simulink subsystem "EoM_Euler6DoF"  (R2024b)
settings: Solver=VariableStepAuto  StartTime=0.0  StopTime=10.0  RelTol=1e-3
undefined symbols (not defined in the file or in its folder): com_error, inertia_error, mass_error, vehicle
settings Model: Creator=thatf  LastModifiedBy=ishkr

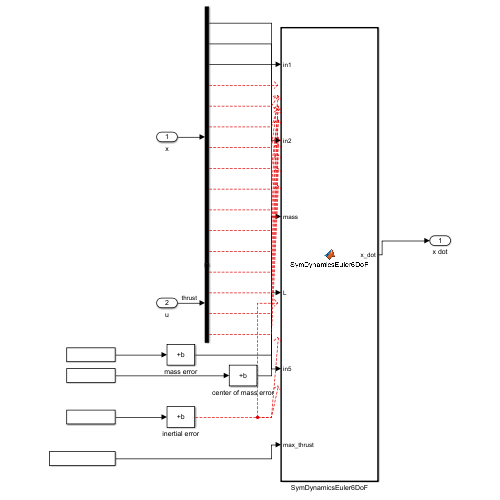
[thumbnail: Simulink's stored preview of the top-level diagram]
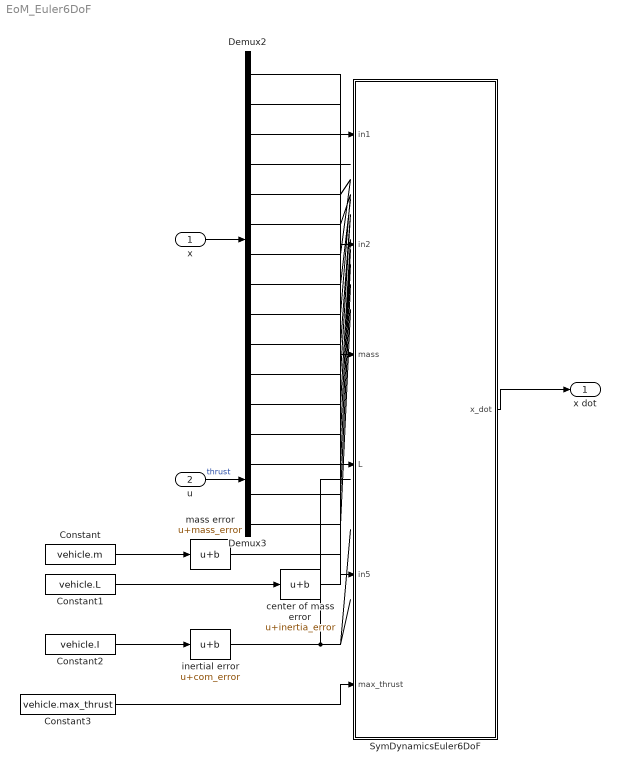
== system EoM_Euler6DoF ==
  x : Inport
  u : Inport  Port=2
  Constant : Constant  Value=vehicle.m
  Constant1 : Constant  Value=vehicle.L
  Constant2 : Constant  Value=vehicle.I
  Constant3 : Constant  Value=vehicle.max_thrust
  Demux2 : Demux  Outputs=dof.nx
  Demux3 : Demux  Outputs=dof.nu
  SymDynamicsEuler6DoF : MATLAB Function  TreatAsAtomicUnit=on
  center of mass error : Bias  Bias=inertia_error  SaturateOnIntegerOverflow=off
  inertial error : Bias  Bias=com_error  SaturateOnIntegerOverflow=off
  mass error : Bias  Bias=mass_error  SaturateOnIntegerOverflow=off
  x dot : Outport
  wires:
  x/1 -> Demux2/1
  Constant1/1 -> center of mass error/1
  Constant2/1 -> inertial error/1
  SymDynamicsEuler6DoF/1(x_dot) -> x dot/1
  u/1 -> Demux3/1  "thrust"
  mass error/1 -> SymDynamicsEuler6DoF/3(mass)
  Constant/1 -> mass error/1
  center of mass error/1 -> SymDynamicsEuler6DoF/4(L)
  Demux3/1 -> ?
  Demux2/11 -> ?
  Demux2/10 -> ?
  Demux2/9 -> ?
  Demux2/8 -> ?
  Demux2/1 -> SymDynamicsEuler6DoF/1(in1)
  Demux2/2 -> SymDynamicsEuler6DoF/2(in2)
  Demux2/3 -> SymDynamicsEuler6DoF/5(in5)
  Demux2/4 -> ?
  Demux2/5 -> ?
  Demux2/6 -> ?
  Demux2/7 -> ?
  Demux3/2 -> ?
  Demux3/3 -> ?
  Constant3/1 -> SymDynamicsEuler6DoF/6(max_thrust)
  Demux2/12 -> ?
  Demux3/4 -> ?
  inertial error/1 -> ?

== matlab function EoM_Euler6DoF/SymDynamicsEuler6DoF ==
  data: in1 input; x_dot output; in2 input; mass input; L input; in5 input; max_thrust input
function x_dot = SymDynamicsEuler6DoF(in1,in2,mass,L,in5,max_thrust)
%#codegen

%    This function was generated by the Symbolic Math Toolbox version 24.2.
%    05-Apr-2025 14:57:34

% in1 = complex(in1);  % if required to enforce complex operations
% in2 = complex(in2);  % if required to enforce complex operations
% mass = complex(mass);  % if required to enforce complex operations
% L = complex(L);  % if required to enforce complex operations
% in5 = complex(in5);  % if required to enforce complex operations
% max_thrust = complex(max_thrust);  % if required to enforce complex operations
I1 = in5(1,:);
I2 = in5(2,:);
I3 = in5(3,:);
T1 = in2(1,:);
T2 = in2(2,:);
T3 = in2(3,:);
gamma1 = in2(4,:);
theta1 = in1(7,:);
theta2 = in1(8,:);
theta3 = in1(9,:);
v1 = in1(4,:);
v2 = in1(5,:);
v3 = in1(6,:);
w1 = in1(10,:);
w2 = in1(11,:);
w3 = in1(12,:);
t2 = cos(gamma1);
t3 = cos(theta1);
t4 = cos(theta2);
t5 = cos(theta3);
t6 = sin(theta1);
t7 = sin(theta2);
t8 = sin(theta3);
t9 = -I3;
t10 = 1.0./mass;
t11 = 1.0./t7;
mt1 = [v1;v2;v3;t2.*t10.*(T1.*max_thrust.*t4+T3.*max_thrust.*t5.*t7+T2.*max_thrust.*t7.*t8);t2.*t10.*(T2.*max_thrust.*(t3.*t5-t4.*t6.*t8)-T3.*max_thrust.*(t3.*t8+t4.*t5.*t6)+T1.*max_thrust.*t6.*t7);-t2.*t10.*(-T2.*max_thrust.*(t5.*t6+t3.*t4.*t8)+T3.*max_thrust.*(t6.*t8-t3.*t4.*t5)+T1.*max_thrust.*t3.*t7)-9.81e+2./1.0e+2;t5.*t11.*w3+t8.*t11.*w2;t5.*w2-t8.*w3;w1-t4.*t5.*t11.*w3-t4.*t8.*t11.*w2;(sin(gamma1).*sqrt(abs(T1.*max_thrust).^2+abs(T2.*max_thrust).^2+abs(T3.*max_thrust).^2)+w2.*w3.*(I2+t9))./I1;-(w1.*w3.*(I1+t9)-L.*T3.*max_thrust.*t2)./I2];
mt2 = [(w1.*w2.*(I1-I2)-L.*T2.*max_thrust.*t2)./I3];
x_dot = [mt1;mt2];
end
